simulink library "Atmosphere_Library"  (R2021a)
settings: Solver=VariableStepAuto  StartTime=0.0  StopTime=10.0  RelTol=1e-3
settings Model: Creator=prave  LastModifiedBy=prave

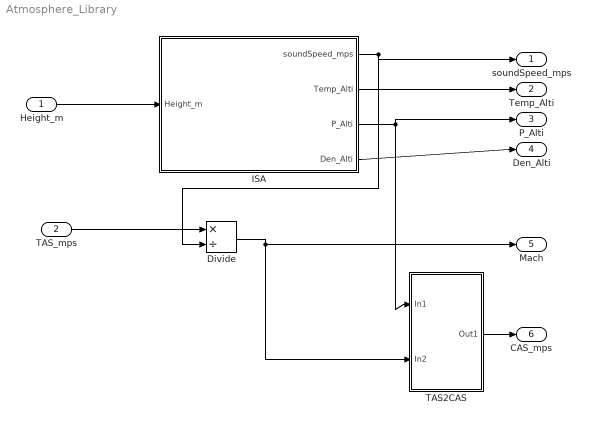
== system Atmosphere_Library ==
  Height_m : Inport
  TAS_mps : Inport  Port=2
  Divide : Product  Inputs=*/
  ISA : Subsystem
  TAS2CAS : Subsystem
  soundSpeed_mps : Outport
  Temp_Alti : Outport  Port=2
  P_Alti : Outport  Port=3
  Den_Alti : Outport  Port=4
  Mach : Outport  Port=5
  CAS_mps : Outport  Port=6
  wires:
  Height_m/1 -> ISA/1(Height_m)
  ISA/1(soundSpeed_mps) -> soundSpeed_mps/1, Divide/2
  ISA/2(Temp_Alti) -> Temp_Alti/1
  ISA/3(P_Alti) -> P_Alti/1, TAS2CAS/1(In1)
  ISA/4(Den_Alti) -> Den_Alti/1
  TAS_mps/1 -> Divide/1
  Divide/1 -> TAS2CAS/2(In2), Mach/1
  TAS2CAS/1(Out1) -> CAS_mps/1

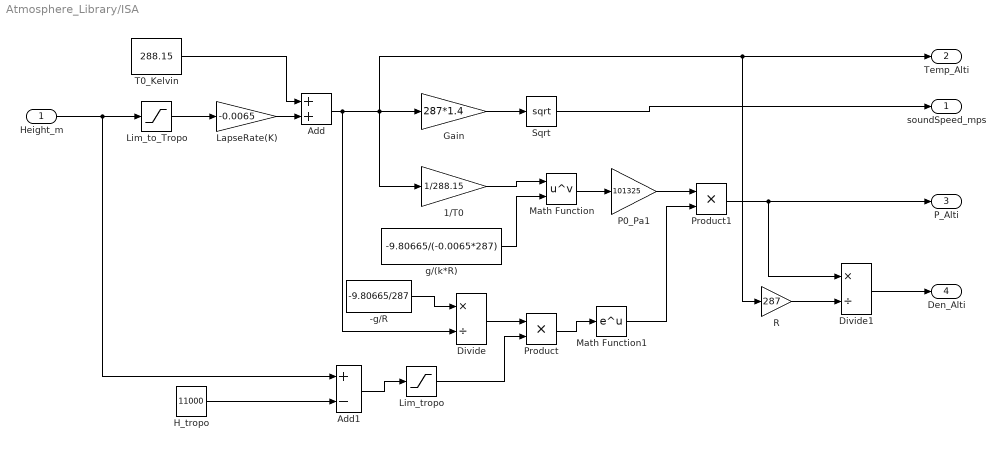
== system Atmosphere_Library/ISA ==
  Height_m : Inport
  -g/R : Constant  Value=-9.80665/287
  1/T0 : Gain  Gain=1/288.15
  Add : Sum
  Add1 : Sum  Inputs=+-
  Divide : Product  Inputs=*/
  Divide1 : Product  Inputs=*/
  Gain : Gain  Gain=287*1.4
  H_tropo : Constant  Value=11000
  LapseRate(K) : Gain  Gain=-0.0065
  Lim_to_Tropo : Saturate  UpperLimit=11000  LowerLimit=0
  Lim_tropo : Saturate  UpperLimit=inf  LowerLimit=0
  Math Function : Math  Operator=pow  SaturateOnIntegerOverflow=on
  Math Function1 : Math  SaturateOnIntegerOverflow=on
  P0_Pa1 : Gain  Gain=101325
  Product : Product
  Product1 : Product
  R : Gain  Gain=287
  Sqrt : Sqrt  SaturateOnIntegerOverflow=on
  T0_Kelvin : Constant  Value=288.15
  g/(k*R) : Constant  Value=-9.80665/(-0.0065*287)
  soundSpeed_mps : Outport
  Temp_Alti : Outport  Port=2
  P_Alti : Outport  Port=3
  Den_Alti : Outport  Port=4
  wires:
  Height_m/1 -> Add1/1, Lim_to_Tropo/1
  P0_Pa1/1 -> Product1/1
  Add1/1 -> Lim_tropo/1
  Divide1/1 -> Den_Alti/1
  H_tropo/1 -> Add1/2
  Add/1 -> 1/T0/1, Temp_Alti/1, R/1, Gain/1, Divide/2
  Math Function1/1 -> Product1/2
  -g/R/1 -> Divide/1
  Gain/1 -> Sqrt/1
  T0_Kelvin/1 -> Add/1
  Divide/1 -> Product/1
  Product1/1 -> P_Alti/1, Divide1/1
  1/T0/1 -> Math Function/1
  LapseRate(K)/1 -> Add/2
  Lim_to_Tropo/1 -> LapseRate(K)/1
  R/1 -> Divide1/2
  Math Function/1 -> P0_Pa1/1
  g/(k*R)/1 -> Math Function/2
  Lim_tropo/1 -> Product/2
  Product/1 -> Math Function1/1
  Sqrt/1 -> soundSpeed_mps/1

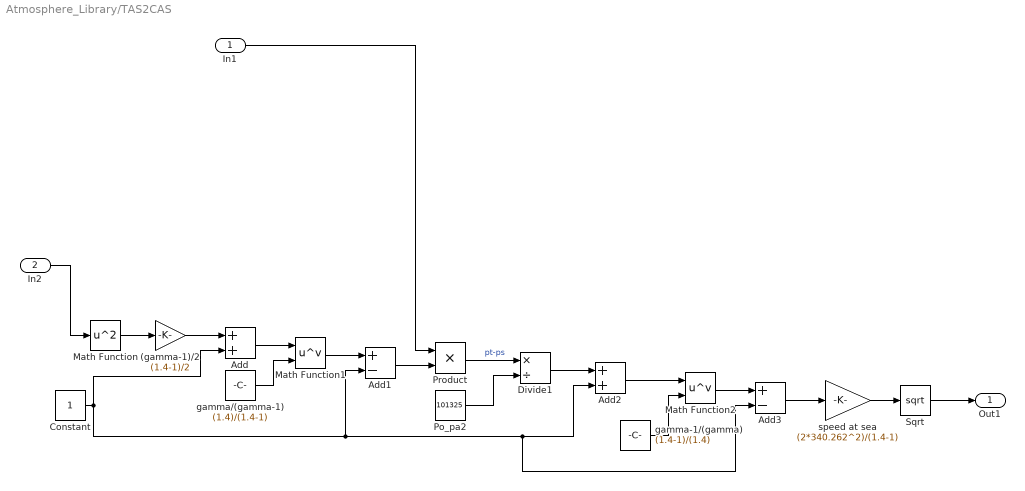
== system Atmosphere_Library/TAS2CAS ==
  In1 : Inport
  In2 : Inport  Port=2
  (gamma-1)/2 : Gain  Gain=(1.4-1)/2
  Add : Sum
  Add1 : Sum  Inputs=+-
  Add2 : Sum
  Add3 : Sum  Inputs=+-
  Constant : Constant
  Divide1 : Product  Inputs=*/
  Math Function : Math  Operator=square  SaturateOnIntegerOverflow=on
  Math Function1 : Math  Operator=pow  SaturateOnIntegerOverflow=on
  Math Function2 : Math  Operator=pow  SaturateOnIntegerOverflow=on
  Po_pa2 : Constant  Value=101325
  Product : Product
  Sqrt : Sqrt  SaturateOnIntegerOverflow=on
  gamma-1/(gamma) : Constant  Value=(1.4-1)/(1.4)
  gamma/(gamma-1) : Constant  Value=(1.4)/(1.4-1)
  speed at sea : Gain  Gain=(2*340.262^2)/(1.4-1)
  Out1 : Outport
  wires:
  Sqrt/1 -> Out1/1
  Math Function1/1 -> Add1/1
  Math Function2/1 -> Add3/1
  speed at sea/1 -> Sqrt/1
  gamma-1/(gamma)/1 -> Math Function2/2
  Constant/1 -> Add/2, Add3/2, Add2/2, Add1/2
  gamma/(gamma-1)/1 -> Math Function1/2
  Math Function/1 -> (gamma-1)/2/1
  Add/1 -> Math Function1/1
  Po_pa2/1 -> Divide1/2
  Divide1/1 -> Add2/1
  Add3/1 -> speed at sea/1
  Add2/1 -> Math Function2/1
  (gamma-1)/2/1 -> Add/1
  Add1/1 -> Product/2
  Product/1 -> Divide1/1  "pt-ps"
  In2/1 -> Math Function/1
  In1/1 -> Product/1
